simulink model "DSM_SIM_R2013b"  (R2013b)
settings: Solver=ode45  StartTime=0.0  StopTime=1.0  RelTol=1e-3
values from neighbouring files (symbols this model uses):
  A = 0.5*(nLev-1)    (= 0.5)    [Model3.m]
  ftest = 9e3    (= 9000)    [Model3.m]    (also in Model3_LTE.m = 2250)
  Ts = 1/Fs    (= 2.03450520833e-06)    [Model3.m]    (also in Model3_LTE.m = 1/Fs)
libraries: xbsIndex_r4 x14
settings Model: Creator=o_cotte  LastModifiedBy=o_cotte

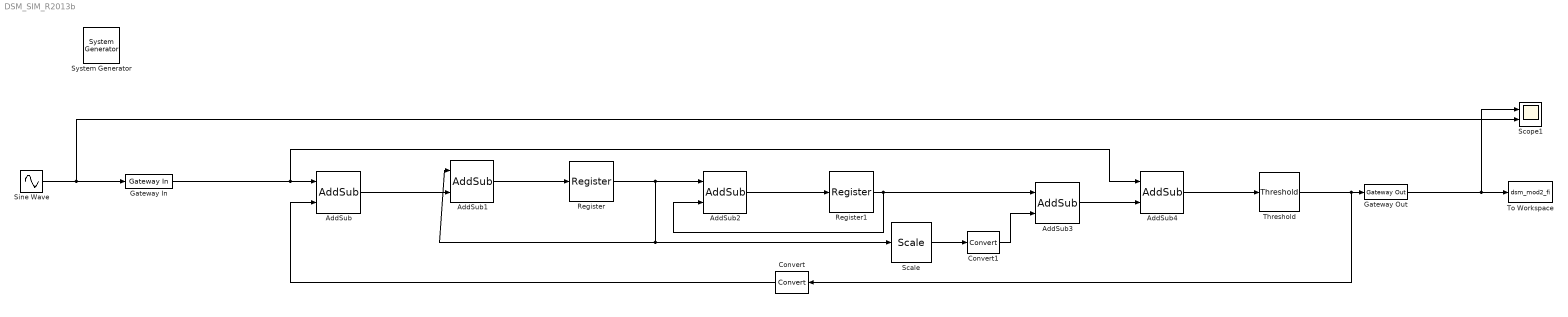
== system DSM_SIM_R2013b ==
  " System Generator" : xbsIndex_r4/ System Generator  Tag=genX  xilinxfamily=spartan6  part=xc6slx45  speed=-2  package=csg324  synthesis_tool=XST  clock_wrapper=Clock Enables  directory=./netlist  proj_type=Project Navigator  Synth_file=XST Defaults  Impl_file=ISE Defaults  testbench=off  simulink_period=Ts  sysclk_period=10  dcm_input_clock_period=10  incr_netlist=off  trim_vbits=Everywhere in SubSystem  dbl_ovrd=According to Block Masks  core_generation=According to Block Masks  run_coregen=off  deprecated_control=off  eval_field=0  block_type=sysgen
  AddSub : xbsIndex_r4/AddSub  mode=Subtraction  use_carryin=off  use_carryout=off  en=off  latency=0  precision=User Defined  arith_type="Signed  (2's comp)"  n_bits=36  bin_pt=32  quantization=Truncate  overflow=Saturate  dbl_ovrd=off  use_behavioral_HDL=off  hw_selection=Fabric  pipelined=off  block_type=addsub
  AddSub{1..4} (4 alike) : xbsIndex_r4/AddSub  mode=Addition  use_carryin=off  use_carryout=off  en=off  latency=0  precision=User Defined  arith_type="Signed  (2's comp)"  n_bits=36  bin_pt=32  quantization=Truncate  overflow=Saturate  dbl_ovrd=off  use_behavioral_HDL=off  hw_selection=Fabric  pipelined=off  block_type=addsub
  Convert : xbsIndex_r4/Convert  gui_display_data_type=Fixed-point  arith_type="Signed  (2's comp)"  n_bits=36  bin_pt=32  float_type=Single  exp_bits=8  fraction_bits=24  quantization=Truncate  overflow=Wrap  en=off  latency=0  dbl_ovrd=off  pipeline=off  block_type=convert
  Convert1 : xbsIndex_r4/Convert  gui_display_data_type=Fixed-point  arith_type="Signed  (2's comp)"  n_bits=36  bin_pt=32  float_type=Single  exp_bits=8  fraction_bits=24  quantization=Truncate  overflow=Wrap  en=off  latency=0  dbl_ovrd=off  pipeline=off  block_type=convert
  Gateway In : xbsIndex_r4/Gateway In  gui_display_data_type=Fixed-point  arith_type="Signed  (2's comp)"  n_bits=36  bin_pt=32  preci_type=Single  exp_width=8  frac_width=24  quantization="Round  (unbiased: +/- Inf)"  overflow=Saturate  period=Ts  dbl_ovrd=off  timing_constraint=None  locs_specified=off  LOCs={}  UseAsADC=off  ADCChannel='1'  inherit_from_input=off  hdl_port=on  block_type=gatewayin
  Gateway Out : xbsIndex_r4/Gateway Out  inherit_from_input=on  hdl_port=on  timing_constraint="Data Rate;  Set 'FAST' Attribute"  locs_specified=off  LOCs={}  UseAsDAC=off  DACChannel='1'  block_type=gatewayout
  Register : xbsIndex_r4/Register  init=0  rst=off  en=off  dbl_ovrd=off  block_type=register
  Register1 : xbsIndex_r4/Register  init=0  rst=off  en=off  dbl_ovrd=off  block_type=register
  Scale : xbsIndex_r4/Scale  scale_factor=1  dbl_ovrd=off  block_type=scale
  Scope1 : Scope  NumInputPorts=2
      settings: TickLabels=on  ShowLegends=on  TimeRange=1  YMin=-1~-0.5  YMax=1~0.5
  Sine Wave : Sin  Amplitude=A  Frequency=ftest  SampleTime=Ts
  Threshold : xbsIndex_r4/Threshold  en=off  latency=0  dbl_ovrd=off  block_type=sgn
      settings: infoedit="Presents -1 as output if input is negative; otherwise presents 1.  Output is a two bit signed number."
  To Workspace : ToWorkspace  VariableName=dsm_mod2_fi  SampleTime=-1
  wires:
  AddSub/1 -> AddSub1/2
  AddSub1/1 -> Register/1
  Register/1 -> AddSub2/1, AddSub1/1, Scale/1
  AddSub2/1 -> Register1/1
  Register1/1 -> AddSub3/1, AddSub2/2
  Sine Wave/1 -> Gateway In/1, Scope1/2
  AddSub3/1 -> AddSub4/2
  AddSub4/1 -> Threshold/1
  Threshold/1 -> Convert/1, Gateway Out/1
  Gateway Out/1 -> To Workspace/1, Scope1/1
  Convert/1 -> AddSub/2
  Scale/1 -> Convert1/1
  Convert1/1 -> AddSub3/2
  Gateway In/1 -> AddSub4/1, AddSub/1
